simulink model "angelbot_ROScommand"  (R2015b)
settings: Solver=FixedStepAuto  StartTime=0.0  StopTime=inf  FixedStep=0.1  RelTol=1e-3
undefined symbols (not defined in the file or in its folder): Angular, Linear
libraries: robotlib x10, realtime_pacer_lib x2
settings Model: Creator=root  LastModifiedBy=shangwei

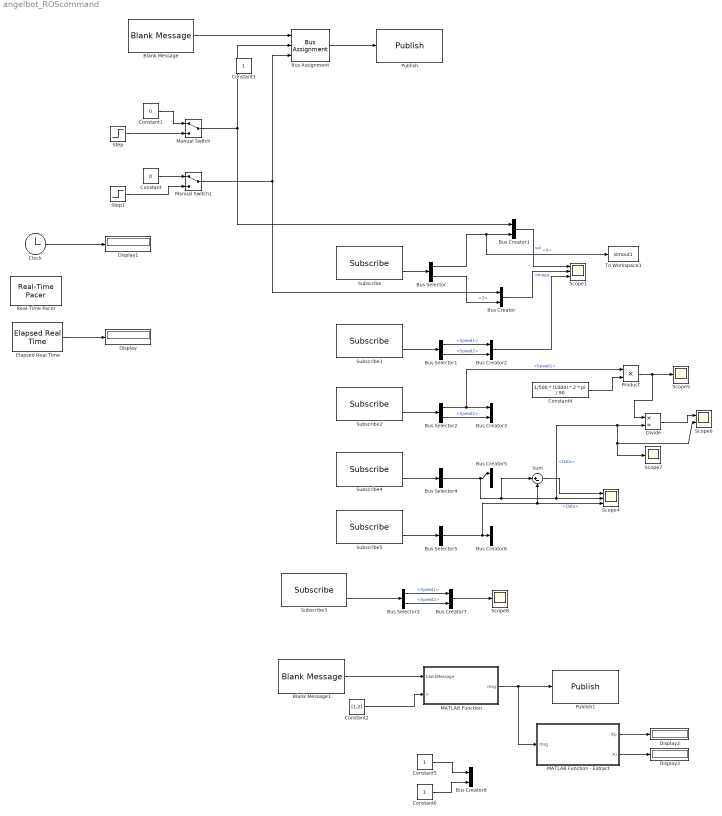
== system angelbot_ROScommand ==
  Blank Message : robotlib/Blank Message  SourceLibraryInfo=This block requires Robotics System Toolbox  messageType=geometry_msgs/Twist  SampleTime=inf
  Blank Message1 : robotlib/Blank Message  SourceLibraryInfo=This block requires Robotics System Toolbox  messageType=std_msgs/Float64MultiArray  SampleTime=inf
  Bus Assignment : BusAssignment  AssignedSignals=Linear.X,Angular.Z
  Bus Creator{,1..3,5,7..8} (7 alike) : BusCreator  Inputs=2
  Bus Creator6 : BusCreator  Inputs=1
  Bus Selector : BusSelector  OutputSignals=Linear.X,Angular.Z
  Bus Selector1 : BusSelector  OutputSignals=Speed1,Speed2
  Bus Selector2 : BusSelector  OutputSignals=Speed1,Speed2
  Bus Selector3 : BusSelector  OutputSignals=Speed1,Speed2
  Bus Selector4 : BusSelector  OutputSignals=Data
  Bus Selector5 : BusSelector  OutputSignals=Data
  Clock : Clock
  Constant : Constant  Value=0  OutDataTypeStr=double  SampleTime=-1
  Constant1 : Constant  Value=0  OutDataTypeStr=double  SampleTime=-1
  Constant2 : Constant  Value=[1,2]
  Constant4 : Constant  Value=1/500 * (1000) * 2 * pi / 90  OutDataTypeStr=double  SampleTime=-1
  Constant5 : Constant  OutDataTypeStr=uint32
  Constant6 : Constant  OutDataTypeStr=uint32
  Display{,1..3} (4 alike) : Display
  Divide : Product  Inputs=*/
  Elapsed Real Time : realtime_pacer_lib/Elapsed Real Time
  MATLAB Function : MATLAB Function  TreatAsAtomicUnit=on
  MATLAB Function - Extract : MATLAB Function  TreatAsAtomicUnit=on
  Manual Switch : ManualSwitch
  Manual Switch1 : ManualSwitch
  Product : Product
  Publish : robotlib/Publish  SourceLibraryInfo=This block requires Robotics System Toolbox  topicSource=Select from ROS network  topic=/angelbot/cmd_vel  messageType=geometry_msgs/Twist  messageQueueLength=1
  Publish1 : robotlib/Publish  SourceLibraryInfo=This block requires Robotics System Toolbox  topicSource=Select from ROS network  topic=/angelbot/VelLoopPID  messageType=std_msgs/Float64MultiArray  messageQueueLength=1
  Real-Time Pacer : realtime_pacer_lib/Real-Time Pacer  simTimePerRealTime=1
  Scope1 : Scope  NumInputPorts=3
  Scope4 : Scope  NumInputPorts=3
  Scope5 : Scope
  Scope6 : Scope  NumInputPorts=2
  Scope7 : Scope
  Scope8 : Scope
  Step : Step  Time=0  After=14
  Step1 : Step  Time=0  After=18
  Subscribe : robotlib/Subscribe  SourceLibraryInfo=This block requires Robotics System Toolbox  topicSource=Select from ROS network  topic=/angelbot/feedbackVel  messageType=geometry_msgs/Twist  sampleTime=-1  messageQueueLength=1
  Subscribe1 : robotlib/Subscribe  SourceLibraryInfo=This block requires Robotics System Toolbox  topicSource=Select from ROS network  topic=/angelbot/cmd_wheel_volt  messageType=angelbot/WheelCmd  sampleTime=-1  messageQueueLength=1
  Subscribe2 : robotlib/Subscribe  SourceLibraryInfo=This block requires Robotics System Toolbox  topicSource=Select from ROS network  topic=/angelbot/WheelInput  messageType=angelbot/WheelCmd  sampleTime=-1  messageQueueLength=1
  Subscribe3 : robotlib/Subscribe  SourceLibraryInfo=This block requires Robotics System Toolbox  topicSource=Select from ROS network  topic=/angelbot/feedback_wheel_angularVel  messageType=angelbot/WheelFb  sampleTime=-1  messageQueueLength=1
  Subscribe4 : robotlib/Subscribe  SourceLibraryInfo=This block requires Robotics System Toolbox  topicSource=Select from ROS network  topic=/ENC_raw  messageType=std_msgs/Int16  sampleTime=-1  messageQueueLength=1
  Subscribe5 : robotlib/Subscribe  SourceLibraryInfo=This block requires Robotics System Toolbox  topicSource=Select from ROS network  topic=/ENCPre_raw  messageType=std_msgs/Int16  sampleTime=-1  messageQueueLength=1
  Sum : Sum  Inputs=|+-
  To Workspace1 : ToWorkspace  VariableName=simout1  SaveFormat=Timeseries  SampleTime=-1
  Constant3 : Constant  IOType=siggen
  wires:
  Bus Assignment/1 -> Publish/1
  Blank Message/1 -> Bus Assignment/1
  Subscribe/2 -> Bus Selector/1
  Bus Selector/1 -> To Workspace1/1, Bus Creator1/2  "<X>"
  Bus Selector/2 -> Bus Creator/2  "<Z>"
  Manual Switch/1 -> Bus Creator1/1, Bus Assignment/2
  Constant1/1 -> Manual Switch/1
  Constant/1 -> Manual Switch1/1
  Manual Switch1/1 -> Bus Assignment/3, Bus Creator/1
  Bus Creator1/1 -> Scope1/1  "vel"
  Bus Creator/1 -> Scope1/2  "omega"
  Step/1 -> Manual Switch/2
  Step1/1 -> Manual Switch1/2
  Elapsed Real Time/1 -> Display/1
  Clock/1 -> Display1/1
  Subscribe1/2 -> Bus Selector1/1
  Bus Selector1/1 -> Bus Creator2/1  "<Speed1>"
  Bus Selector1/2 -> Bus Creator2/2  "<Speed2>"
  Bus Creator2/1 -> Scope1/3
  Subscribe2/2 -> Bus Selector2/1
  Bus Selector2/1 -> Product/1, Bus Creator3/1  "<Speed1>"
  Subscribe3/2 -> Bus Selector3/1
  Bus Selector2/2 -> Bus Creator3/2  "<Speed2>"
  Subscribe4/2 -> Bus Selector4/1
  Bus Selector4/1 -> Sum/1, Scope7/1, Scope6/2, Divide/2, Scope4/2, Bus Creator5/1  "<Data>"
  Subscribe5/2 -> Bus Selector5/1
  Bus Selector5/1 -> Sum/2, Scope4/3, Bus Creator6/1  "<Data>"
  Sum/1 -> Scope4/1
  Constant4/1 -> Product/2
  Product/1 -> Divide/1, Scope5/1
  Divide/1 -> Scope6/1
  Bus Selector3/1 -> Bus Creator7/1  "<Speed1>"
  Bus Selector3/2 -> Bus Creator7/2  "<Speed2>"
  Bus Creator7/1 -> Scope8/1
  Constant2/1 -> MATLAB Function/2(u)
  Constant5/1 -> Bus Creator8/1
  Constant6/1 -> Bus Creator8/2
  Blank Message1/1 -> MATLAB Function/1(blankMessage)
  MATLAB Function/1(msg) -> MATLAB Function - Extract/1(msg), Publish1/1
  MATLAB Function - Extract/1(Kp) -> Display2/1
  MATLAB Function - Extract/2(Ki) -> Display3/1

== matlab function angelbot_ROScommand/MATLAB Function ==
  data: blankMessage input; u input; msg output Bus: SL_Bus_angelbot_ROScommand_std_msgs_Float64MultiArray
function msg = assignArrayMessages(blankMessage,u)
%#codegen

% To set datatype of MSG output:
%  1. Create buses for this model: robotics.ros.createSimulinkBus(gcs)
%  1. Click "Edit Data" in  Toolstrip to open "Ports and Data Manager"
%  2. Select MSG and set datatype to "Bus: SL_Bus_<modelname>_<messageType>"
% See: 
% http://www.mathworks.com/help/simulink/ug/create-structures-in-matlab-function-blocks.html

% blankMessage (geometry_msgs/PoseArray) consists of
%          Header: [1x1 Header]
%           Poses: variable-length array of geometry_msgs/Pose
%   Poses_SL_Info: struct with fields CurrentLength, ReceivedLength
%
% Poses is an array of "geometry_msgs/Pose", which consists of
%        Position: [1x1 Point]
%     Orientation: [1x1 Quaternion]
%
% Position is "geometry_msgs/Point", which consists of
%               X: 0
%               Y: 0
%               Z: 0
%
% Orientation is "geometry_msgs/Quaternion", which consists of
%               X: 0
%               Y: 0
%               Z: 0
%               W: 0

% Set the Poses array to have size 2, and modify the first two Pose
% elements

blankMessage.Data_SL_Info.CurrentLength = uint32(2);
blankMessage.Data(1) = u(1);
blankMessage.Data(2) = u(2);

msg = blankMessage;

== matlab function angelbot_ROScommand/MATLAB Function - Extract ==
  data: msg input; Kp output; Ki output
function [Kp,Ki] = extractNestedArrayMessages(msg)
%#codegen

% geometry_msgs/PoseArray consists of
%          Header: [1x1 Header]
%           Poses: [nx1 Pose]

% Poses is an array of "geometry_msgs/Pose", which consists of
%        Position: [1x1 Point]
%     Orientation: [1x1 Quaternion]

% Position is "geometry_msgs/Point", which consists of
%               X: 0
%               Y: 0
%               Z: 0

% Orientation is "geometry_msgs/Quaternion", which consists of
%               X: 0
%               Y: 0
%               Z: 0
%               W: 0

% Extract elements from an array with specified indices (1,2) and extract
% information from those elements
Kp = msg.Data(1);
Ki = msg.Data(2);
